simulink model "Splitter_TestBed_org"  (Simulink 10.0)
settings: Solver=FixedStepDiscrete  StartTime=0.0  StopTime=1  FixedStep=1  RelTol=1e-3  EnableMultiTasking=on
undefined symbols (not defined in the file): MWS
libraries: Lib_Turbo_Splitter_TMATS x1
settings Model: Creator=jwchapm2  LastModifiedBy=bhisma
settings DataIOCC: LimitDataPoints=on
settings OptimizationCC: ExpressionDepthLimit=2147483647
settings DebuggingCC: SolverPrmCheckMsg=warning  StateNameClashWarn=warning
settings GRTTargetCC: GeneratePreprocessorConditionals=Disable all  CombineOutputUpdateFcns=on  GRTInterface=off
settings ConfigComp: CovExternalEMLEnable=off

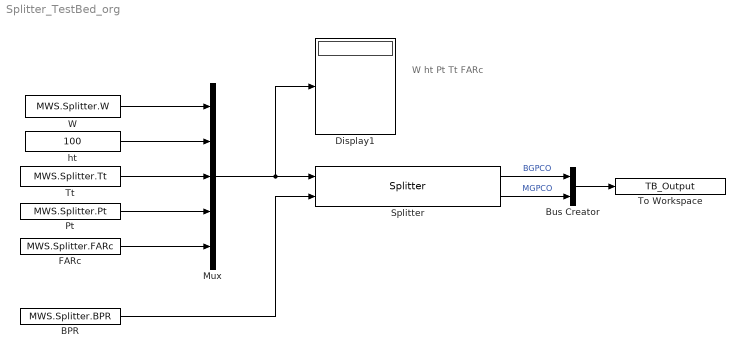
== system Splitter_TestBed_org ==
  note: W
      | ht
      | Pt
      | Tt
      | FARc
  BPR : Constant  Value=MWS.Splitter.BPR
  Bus Creator : BusCreator  Inputs=2
  Display1 : Display
  FARc : Constant  Value=MWS.Splitter.FARc
  Mux : Mux  Inputs=5
  Pt : Constant  Value=MWS.Splitter.Pt
  Splitter : Lib_Turbo_Splitter_TMATS/Splitter
  To Workspace : ToWorkspace  VariableName=TB_Output  SampleTime=-1
  Tt : Constant  Value=MWS.Splitter.Tt
  W : Constant  Value=MWS.Splitter.W
  ht : Constant  Value=100
  wires:
  W/1 -> Mux/1
  FARc/1 -> Mux/5
  Tt/1 -> Mux/3
  Pt/1 -> Mux/4
  Mux/1 -> Splitter/1, Display1/1
  Splitter/1 -> Bus Creator/1  "BGPCO"
  Bus Creator/1 -> To Workspace/1
  ht/1 -> Mux/2
  Splitter/2 -> Bus Creator/2  "MGPCO"
  BPR/1 -> Splitter/2
